simulink model "rtwdemo_pmsmfoc_nn"  (Simulink 7.9)
settings: Solver=FixedStepDiscrete  SolverMode=SingleTasking  StartTime=0.0  StopTime=0.14  FixedStep=ctrlConst.TsHi  RelTol=1e-3
PreLoadFcn:
  | rtwdemo_pmsmfoc_data
undefined symbols (not defined in the file or in its folder): ctrlConst, ctrlParams, DiscIntNeverNeededParam, EnumControllerMode, EnumErrorType
libraries: simulink x15
(part 1 of 2)
Description:
  | Controller Algorithm for Permanent Magnet Synchronous Machine
  | 
  | Specifies controller software component for Permanent Magnet Synchronous Machine (PMSM) using Field-Oriented Control.
  | The sensors bus/structure contains values returned by the Analog to Digital Converter (ADC) and quadrature encoder peripherals.
  | The controller outputs compare values used by the Pulse Width Modulators (PWMs) to generate the phase voltages.
settings Model: MinMaxOverflowLogging=ForceOff  Creator=The MathWorks Inc.  LastModifiedBy=bas  CovHTMLOptions=-aTS=1 -bRG=1 -bTC=1 -hTR=0 -nFC=0 -scm=1 -bcm=1 -xEv=0
settings DataIOCC: ExternalInput=in.motor_on in.command_type in.command_value in.sensors  LimitDataPoints=off  SaveFormat=StructureWithTime  SaveOutput=off  DSMLogging=off  SaveTime=off
settings OptimizationCC: InlineParams=on  UseFloatMulNetSlope=on  UseSpecifiedMinMax=on  InlineInvariantSignals=on  EnhancedBackFolding=on  StrengthReduction=on  ZeroExternalMemoryAtStartup=off  EfficientFloat2IntCast=on  OptimizeModelRefInitCode=on  LifeSpan=1  SimCompilerOptimization=On
settings DebuggingCC: AlgebraicLoopMsg=none  SolverPrmCheckMsg=none  SingleTaskRateTransMsg=error  IntegerOverflowMsg=none  ParameterPrecisionLossMsg=none  UniqueDataStoreMsg=error  AssertControl=DisableAll  ModelReferenceSymbolNameMessage=none
settings HardwareCC: ProdEndianess=LittleEndian  ProdHWDeviceType=Generic->32-bit Embedded Processor
settings ModelReferenceCC: ModelReferenceNumInstancesAllowed=Single
settings RTWCC: SystemTargetFile=nanonote.tlc  TemplateMakefile=nanonote.tmf  Description=Ben NanoNote  GenerateReport=on  RTWVerbose=off  ProcessScript=nanonote_make_rtw_hook  IncludeHyperlinkInReport=on  LaunchReport=on  GenerateTraceInfo=on  GenerateTraceReport=on  GenerateTraceReportSl=on  GenerateTraceReportSf=on  GenerateTraceReportEml=on  GenerateCodeMetricsReport=on  RTWCompilerOptimization=On
settings CodeAppCC: IgnoreCustomStorageClasses=off  IgnoreTestpoints=on  MATLABFcnDesc=on  CustomSymbolStrGlobalVar=$N$M  CustomSymbolStrType=$N$M  CustomSymbolStrFcn=$N$M$F  CustomSymbolStrFcnArg=$N$M  CustomSymbolStrBlkIO=$N$M  CustomSymbolStrMacro=$N$M  MATLABSourceComments=on  ReqsInCode=on
settings STFCustomTargetCC: CodeReplacementLibrary=ANSI_C  CombineOutputUpdateFcns=on  ERTCustomFileBanners=on  SupportContinuousTime=off  SupportNonInlinedSFcns=off  GRTInterface=off  SystemTargetFile=nanonote.tlc
settings ERTTargetCC: CodeReplacementLibrary=ANSI_C  MultiwordLength=2048  ParMdlRefBuildCompliant=off  CompOptLevelCompliant=off  ConcurrentExecutionCompliant=off  ERTFirstTimeCompliant=off  ModelStepFunctionPrototypeControlCompliant=off  CPPClassGenCompliant=off  InlinedParameterPlacement=NonHierarchical  ERTCustomFileTemplate=nanonote_srmain.tlc  ConvertIfToSwitch=off  SuppressUnreachableDefaultCases=off
settings CustomProperty: Value=on
settings ConfigurationSet: Description=SimMechanics 2G
settings ConfigComp: Description=Design Verifier Custom Configuration Component  DVMode=DesignErrorDetection  DVOutputDir=Work/sldv_output/$ModelName$  DVMaxTestCaseSteps=500  DVTestSuiteOptimization=CombinedObjectives (Nonlinear Extended)  DVDesignMinMaxCheck=on  DVSaveReport=on

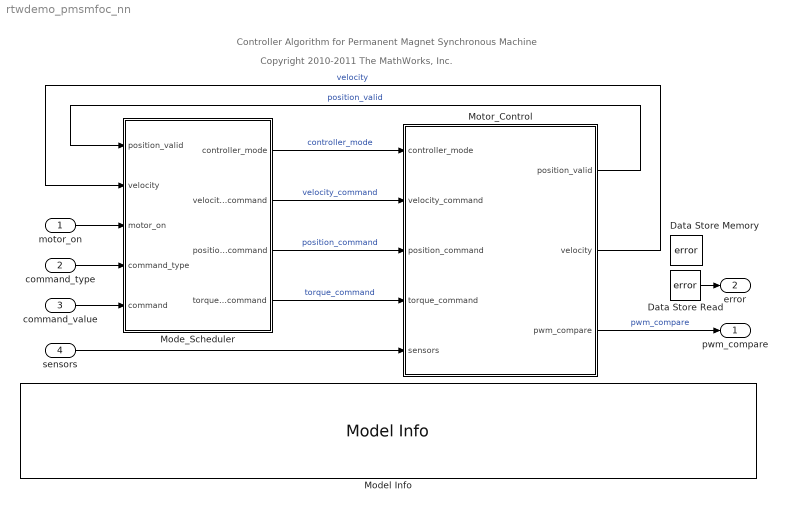
== system rtwdemo_pmsmfoc_nn ==
  note: Controller Algorithm for Permanent Magnet Synchronous Machine
  note: Copyright 2010-2011 The MathWorks, Inc.
  motor_on : Inport  OutDataTypeStr=uint16
  command_type : Inport  Port=2  OutDataTypeStr=Enum: EnumCommandType  Interpolate=off
  command_value : Inport  Port=3  OutDataTypeStr=single  Interpolate=off
  sensors : Inport  Port=4  OutDataTypeStr=Bus: SENSORS_STRUCT  PortDimensions=1  SampleTime=ctrlConst.TsHi  Interpolate=off  BusOutputAsStruct=on
  Data Store Memory : DataStoreMemory  DataStoreName=error  WriteAfterWriteMsg=warning  InitialValue=EnumErrorType.NoError  OutDataTypeStr=Enum: EnumErrorType
  Data Store Read : DataStoreRead  DataStoreName=error  SampleTime=ctrlConst.TsHi
  Mode_Scheduler : Subsystem
      mask Display: fprintf('Mode\nScheduler')
  Model Info : simulink/Model-Wide Utilities/Model Info  InitialBlockCM=None  BlockCM=None  Frame=on  DisplayStringWithTags=Model Description: %<Description>  HorizontalTextAlignment=Left  LeftAlignmentValue=0.02  SourceBlockDiagram=rtwdemo_pmsmfoc_nn  TagMaxNumber=20
  Motor_Control : Subsystem
      settings: RTWSystemCode=Function  RTWFcnNameOpts=Use subsystem name
      mask Display: fprintf('Motor\nControl')
  pwm_compare : Outport
  error : Outport  Port=2
  wires:
  motor_on/1 -> Mode_Scheduler/3(motor_on)
  sensors/1 -> Motor_Control/5(sensors)
  command_type/1 -> Mode_Scheduler/4(command_type)
  Motor_Control/3(pwm_compare) -> pwm_compare/1  "pwm_compare"
  Motor_Control/1(position_valid) -> Mode_Scheduler/1(position_valid)  "position_valid"
  command_value/1 -> Mode_Scheduler/5(command)
  Mode_Scheduler/1(controller_mode) -> Motor_Control/1(controller_mode)  "controller_mode"
  Mode_Scheduler/2(velocity_command) -> Motor_Control/2(velocity_command)  "velocity_command"
  Mode_Scheduler/3(position_command) -> Motor_Control/3(position_command)  "position_command"
  Mode_Scheduler/4(torque_command) -> Motor_Control/4(torque_command)  "torque_command"
  Motor_Control/2(velocity) -> Mode_Scheduler/2(velocity)  "velocity"
  Data Store Read/1 -> error/1

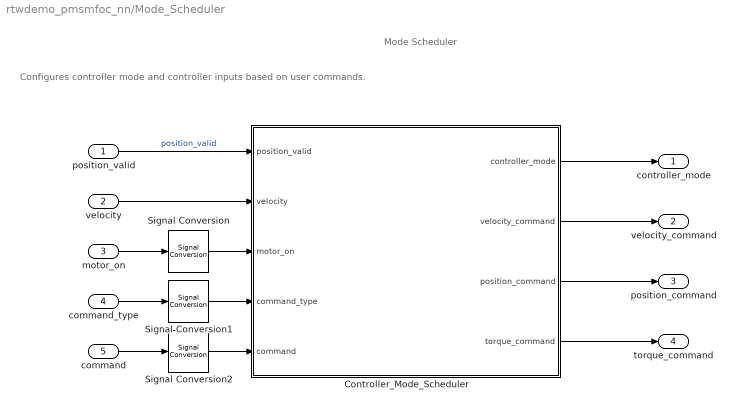
== system rtwdemo_pmsmfoc_nn/Mode_Scheduler ==
  note: Configures controller mode and controller inputs based on user commands.
  note: Mode Scheduler
  position_valid : Inport
  velocity : Inport  Port=2
  motor_on : Inport  Port=3
  command_type : Inport  Port=4
  command : Inport  Port=5
  Controller_Mode_Scheduler : Stateflow chart  TreatAsAtomicUnit=on
  Signal Conversion : SignalConversion  OverrideOpt=on
  Signal Conversion1 : SignalConversion  OverrideOpt=on
  Signal Conversion2 : SignalConversion  OverrideOpt=on
  controller_mode : Outport
  velocity_command : Outport  Port=2
  position_command : Outport  Port=3
  torque_command : Outport  Port=4
  wires:
  position_valid/1 -> Controller_Mode_Scheduler/1(position_valid)  "position_valid"
  Controller_Mode_Scheduler/1(controller_mode) -> controller_mode/1
  velocity/1 -> Controller_Mode_Scheduler/2(velocity)
  Controller_Mode_Scheduler/2(velocity_command) -> velocity_command/1
  motor_on/1 -> Signal Conversion/1
  Controller_Mode_Scheduler/3(position_command) -> position_command/1
  command_type/1 -> Signal Conversion1/1
  Controller_Mode_Scheduler/4(torque_command) -> torque_command/1
  command/1 -> Signal Conversion2/1
  Signal Conversion/1 -> Controller_Mode_Scheduler/3(motor_on)
  Signal Conversion1/1 -> Controller_Mode_Scheduler/4(command_type)
  Signal Conversion2/1 -> Controller_Mode_Scheduler/5(command)

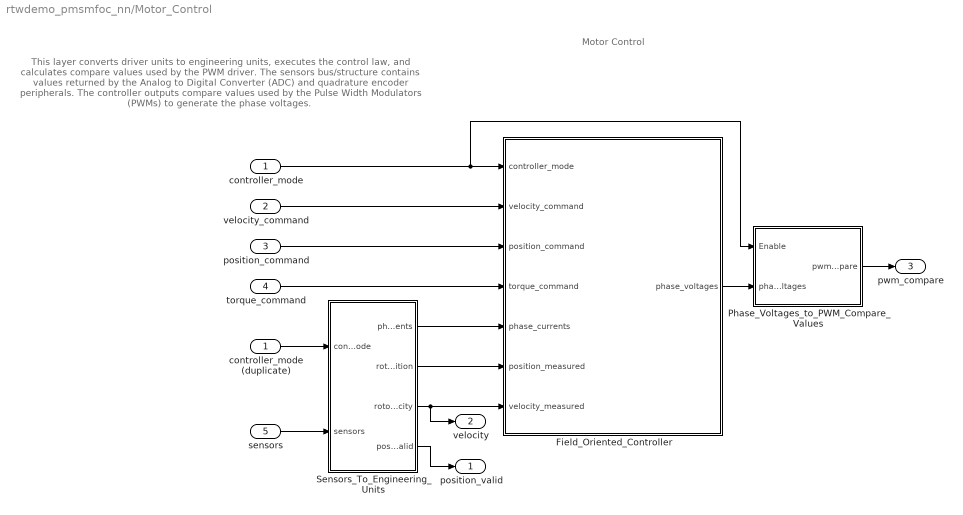
== system rtwdemo_pmsmfoc_nn/Motor_Control ==
  note: This layer converts driver units to engineering units, executes the control law, and calculates compare values used by the PWM driver.
      | The sensors bus/structure contains values returned by the Analog to Digital Converter (ADC) and quadrature encoder peripherals.
      | The controller outputs compare values used by the Pulse Width Modulators (PWMs) to generate the phase voltages.
  note: Motor Control
  controller_mode : Inport
  velocity_command : Inport  Port=2
  position_command : Inport  Port=3
  torque_command : Inport  Port=4
  sensors : Inport  Port=5
  Field_Oriented_Controller : Subsystem
  Phase_Voltages_to_PWM_Compare_Values : Subsystem
      mask Display: fprintf('Phase Voltages\nto PWM\nCompare Values');
  Sensors_To_Engineering_Units : Subsystem
      mask Display: fprintf('Sensors\nto\nEngineering\nUnits')
  controller_mode (duplicate) : InportShadow  Port=1
  position_valid : Outport
  velocity : Outport  Port=2
  pwm_compare : Outport  Port=3
  wires:
  Phase_Voltages_to_PWM_Compare_Values/1(pwm_compare) -> pwm_compare/1
  Field_Oriented_Controller/1(phase_voltages) -> Phase_Voltages_to_PWM_Compare_Values/2(phase_voltages)
  Sensors_To_Engineering_Units/1(phase_currents) -> Field_Oriented_Controller/5(phase_currents)
  controller_mode/1 -> Field_Oriented_Controller/1(controller_mode), Phase_Voltages_to_PWM_Compare_Values/1(Enable)
  sensors/1 -> Sensors_To_Engineering_Units/2(sensors)
  Sensors_To_Engineering_Units/4(position_valid) -> position_valid/1
  Sensors_To_Engineering_Units/3(rotor_velocity) -> velocity/1, Field_Oriented_Controller/7(velocity_measured)
  velocity_command/1 -> Field_Oriented_Controller/2(velocity_command)
  position_command/1 -> Field_Oriented_Controller/3(position_command)
  torque_command/1 -> Field_Oriented_Controller/4(torque_command)
  Sensors_To_Engineering_Units/2(rotor_position) -> Field_Oriented_Controller/6(position_measured)
  controller_mode (duplicate)/1 -> Sensors_To_Engineering_Units/1(controller_mode)

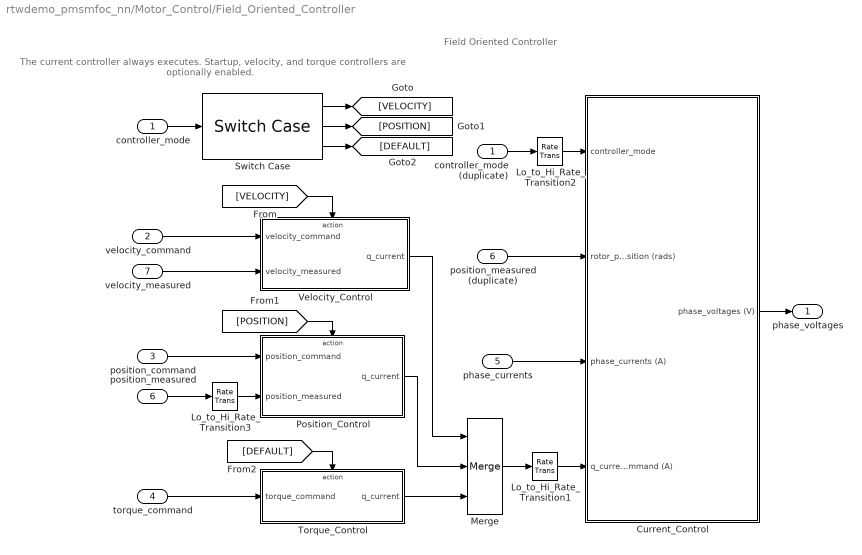
== system rtwdemo_pmsmfoc_nn/Motor_Control/Field_Oriented_Controller ==
  note: The current controller always executes. Startup, velocity, and torque controllers are optionally enabled.
  note: Field Oriented Controller
  controller_mode : Inport
  velocity_command : Inport  Port=2
  position_command : Inport  Port=3
  torque_command : Inport  Port=4
  phase_currents : Inport  Port=5
  position_measured : Inport  Port=6
  velocity_measured : Inport  Port=7
  Current_Control : Subsystem
  Lo_to_Hi_Rate_Transition1 : RateTransition  Integrity=off  OutPortSampleTimeMultiple=25  OutPortSampleTime=ctrlConst.TsHi
  Lo_to_Hi_Rate_Transition2 : RateTransition  Integrity=off  OutPortSampleTimeMultiple=25  OutPortSampleTime=ctrlConst.TsHi
  Lo_to_Hi_Rate_Transition3 : RateTransition  Integrity=off  OutPortSampleTimeMultiple=25  OutPortSampleTime=ctrlConst.TsLo
  Merge : Merge  Inputs=3
  Position_Control : Subsystem  TreatAsAtomicUnit=on
  Switch Case : SwitchCase  CaseConditions={EnumControllerMode.VelocityControl,EnumControllerMode.PositionControl}
  Torque_Control : Subsystem  TreatAsAtomicUnit=on
  Velocity_Control : Subsystem
  controller_mode (duplicate) : InportShadow  Port=1
  position_measured (duplicate) : InportShadow  Port=6
  phase_voltages : Outport
  wires:
  Current_Control/1(phase_voltages (V)) -> phase_voltages/1
  velocity_measured/1 -> Velocity_Control/2(velocity_measured)
  Position_Control/1(q_current) -> Merge/2
  Velocity_Control/1(q_current) -> Merge/1
  Torque_Control/1(q_current) -> Merge/3
  controller_mode/1 -> Switch Case/1
  Merge/1 -> Lo_to_Hi_Rate_Transition1/1
  phase_currents/1 -> Current_Control/3(phase_currents (A))
  controller_mode (duplicate)/1 -> Lo_to_Hi_Rate_Transition2/1
  velocity_command/1 -> Velocity_Control/1(velocity_command)
  position_measured (duplicate)/1 -> Current_Control/2(rotor_position (rads))
  torque_command/1 -> Torque_Control/1(torque_command)
  position_command/1 -> Position_Control/1(position_command)
  position_measured/1 -> Lo_to_Hi_Rate_Transition3/1
  Switch Case/1 -> [VELOCITY]
  Switch Case/2 -> [POSITION]
  Switch Case/3 -> [DEFAULT]
  [VELOCITY] -> Velocity_Control/Action
  [POSITION] -> Position_Control/Action
  [DEFAULT] -> Torque_Control/Action
  Lo_to_Hi_Rate_Transition3/1 -> Position_Control/2(position_measured)
  Lo_to_Hi_Rate_Transition1/1 -> Current_Control/4(q_current_command (A))
  Lo_to_Hi_Rate_Transition2/1 -> Current_Control/1(controller_mode)

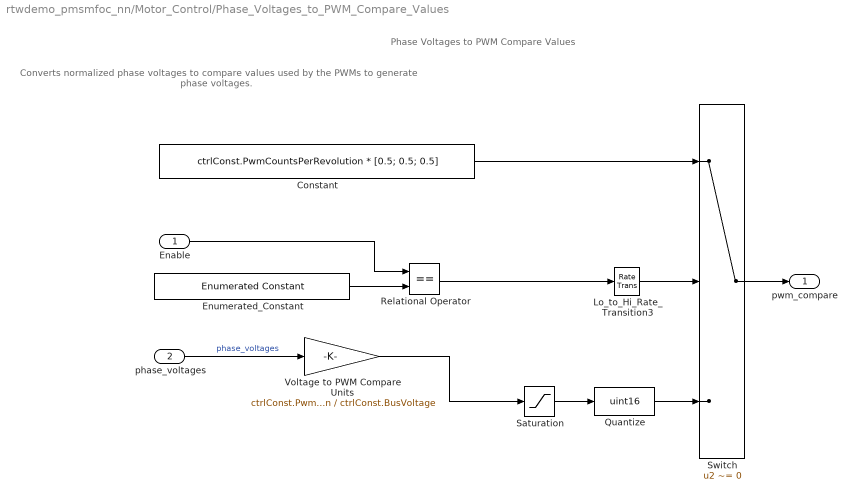
== system rtwdemo_pmsmfoc_nn/Motor_Control/Phase_Voltages_to_PWM_Compare_Values ==
  note: Converts normalized phase voltages to compare values used by the PWMs to generate phase voltages.
  note: Phase Voltages to PWM Compare Values
  Enable : Inport
  phase_voltages : Inport  Port=2
  Constant : Constant  Value=ctrlConst.PwmCountsPerRevolution * [0.5; 0.5; 0.5]  OutDataTypeStr=uint16
  Enumerated_Constant : simulink/Sources/Enumerated Constant  OutDataTypeStr=Enum: EnumControllerMode  Value=EnumControllerMode.StandBy  SampleTime=inf
  Lo_to_Hi_Rate_Transition3 : RateTransition  Deterministic=off  OutPortSampleTimeMultiple=25  OutPortSampleTime=ctrlConst.TsHi
      settings: AttributesFormatString=------------------\nSample Time:\n%<OutPortSampleTime>
  Quantize : DataTypeConversion  OutDataTypeStr=uint16  RndMeth=Simplest
  Relational Operator : RelationalOperator  Operator===  OutDataTypeStr=boolean
  Saturation : Saturate  UpperLimit=ctrlConst.PwmCountsPerRevolution - 1  LowerLimit=0
      settings: AttributesFormatString=--------------------------------\nUpper Limit: %<UpperLimit>\nLower Limit: %<LowerLimit>
  Switch : Switch  Criteria=u2 ~= 0
  Voltage to PWM Compare Units : Gain  Gain=ctrlConst.PwmCountsPerRevolution / ctrlConst.BusVoltage
      settings: AttributesFormatString=----------------------------------------\nGain:\n%<Gain>
  pwm_compare : Outport
  wires:
  phase_voltages/1 -> Voltage to PWM Compare Units/1  "phase_voltages"
  Voltage to PWM Compare Units/1 -> Saturation/1
  Switch/1 -> pwm_compare/1
  Lo_to_Hi_Rate_Transition3/1 -> Switch/2
  Enumerated_Constant/1 -> Relational Operator/2
  Enable/1 -> Relational Operator/1
  Relational Operator/1 -> Lo_to_Hi_Rate_Transition3/1
  Constant/1 -> Switch/1
  Saturation/1 -> Quantize/1
  Quantize/1 -> Switch/3

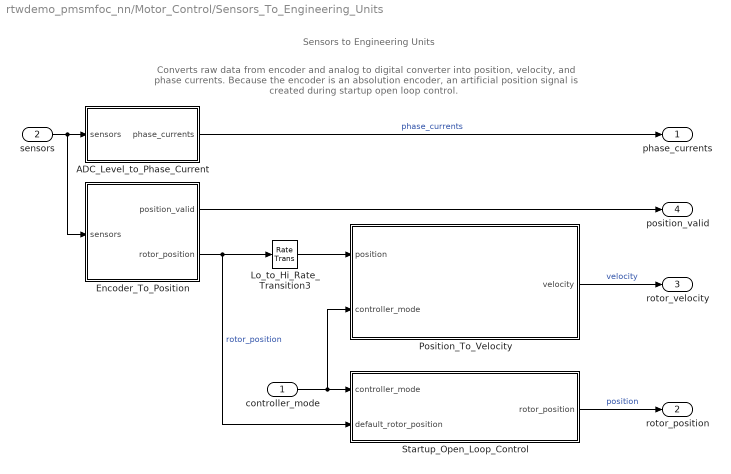
== system rtwdemo_pmsmfoc_nn/Motor_Control/Sensors_To_Engineering_Units ==
  note: Sensors to Engineering Units
  note: Converts raw data from encoder and analog to digital converter into position, velocity, and phase currents.
      | Because the encoder is an absolution encoder, an artificial position signal is created during startup open loop control.
  controller_mode : Inport
  sensors : Inport  Port=2
  ADC_Level_to_Phase_Current : Subsystem
      mask Display: fprintf('ADC Level\nto\nPhase Currents')
  Encoder_To_Position : Subsystem
      mask Display: fprintf('Encoder\nto\nPosition')
  Lo_to_Hi_Rate_Transition3 : RateTransition  Integrity=off  OutPortSampleTimeMultiple=25  OutPortSampleTime=ctrlConst.TsLo
      settings: AttributesFormatString=------------------\nSample Time:\n%<OutPortSampleTime>
  Position_To_Velocity : Subsystem  Variant=on  OverrideUsingVariant=IMPLICIT_WITH_ERROR
  Startup_Open_Loop_Control : Subsystem
      mask Display: fprintf('Startup\nOpen Loop\nControl')
  phase_currents : Outport
  rotor_position : Outport  Port=2
  rotor_velocity : Outport  Port=3
  position_valid : Outport  Port=4
  wires:
  ADC_Level_to_Phase_Current/1(phase_currents) -> phase_currents/1  "phase_currents"
  sensors/1 -> ADC_Level_to_Phase_Current/1(sensors), Encoder_To_Position/1(sensors)
  Position_To_Velocity/1(velocity) -> rotor_velocity/1  "velocity"
  Lo_to_Hi_Rate_Transition3/1 -> Position_To_Velocity/1(position)
  Startup_Open_Loop_Control/1(rotor_position) -> rotor_position/1  "position"
  controller_mode/1 -> Startup_Open_Loop_Control/1(controller_mode), Position_To_Velocity/2(controller_mode)
  Encoder_To_Position/1(position_valid) -> position_valid/1
  Encoder_To_Position/2(rotor_position) -> Startup_Open_Loop_Control/2(default_rotor_position), Lo_to_Hi_Rate_Transition3/1  "rotor_position"

== system rtwdemo_pmsmfoc_nn/Motor_Control/Field_Oriented_Controller/Current_Control ==
  note: Controls stator currents based on transformations between a three-phase phase time and speed dependent system (ABC)
      | and a two coordinate time invariant system (dq).
  note: Current Control
  controller_mode : Inport
  rotor_position (rads) : Inport  Port=2
  phase_currents (A) : Inport  Port=3
  q_current_command (A) : Inport  Port=4
  Current_Controllers : Subsystem  Description=|
      | Linear Current Controllers
      | 
      | PID Blocks used for Control Design of Current Loop controllers.
  Detect_Change : simulink/Logic and Bit Operations/Detect Change  vinit=0  InputProcessing=Inherited  OutDataTypeStr=uint8
  Enum_To_Int : DataTypeConversion  OutDataTypeStr=int16
  Rotation_Coefficients_Sin_Cos : Subsystem
      mask Display: disp('Rotation\nCoefficients\n(sin, cos)')
  Transform_Coordinates_ABC_to_dq : Subsystem
      settings: RTWSystemCode=Function
      mask Display: disp('Transform\nCoordinates\nABC to dq')
  Transform_Coordinates_dq_to_ABC : Subsystem
      settings: RTWSystemCode=Function
      mask Display: disp('Transform\nCoordinates\ndq to ABC')
  phase_voltages (V) : Outport
  wires:
  Current_Controllers/1(dq_axis_voltages (V)) -> Transform_Coordinates_dq_to_ABC/1(dq_voltages)
  phase_currents (A)/1 -> Transform_Coordinates_ABC_to_dq/1(phase_currents)
  Rotation_Coefficients_Sin_Cos/1(sin_cos) -> Transform_Coordinates_dq_to_ABC/2(rotation_coefficients), Transform_Coordinates_ABC_to_dq/2(rotation_coefficients)
  Transform_Coordinates_dq_to_ABC/1(phase_voltages) -> phase_voltages (V)/1
  Transform_Coordinates_ABC_to_dq/1(d_current) -> Current_Controllers/3(d_current_measured (A))
  controller_mode/1 -> Enum_To_Int/1
  rotor_position (rads)/1 -> Rotation_Coefficients_Sin_Cos/1(rotor_position)
  q_current_command (A)/1 -> Current_Controllers/2(q_current_command (A))
  Transform_Coordinates_ABC_to_dq/2(q_current) -> Current_Controllers/4(q_current_measured (A))
  Detect_Change/1 -> Current_Controllers/1(reset_integrators)
  Enum_To_Int/1 -> Detect_Change/1

== system rtwdemo_pmsmfoc_nn/Motor_Control/Field_Oriented_Controller/Position_Control ==
  note: The controller regulates motor position using rotor position feedback compared to a commanded position.
      | The output of the controller is the quadrature-winding current command which is directly proportional to the electromagnetic torque of the motor.
      | Since the motor being controlled is a Permanent Magnet Synchronous Machine, the rotor flux linkage is fixed (determined by the magnets),
      | hence the commanded direct-winding current is always zero.
  note: Position Controller
  position_command : Inport
  position_measured : Inport  Port=2
  Action Port : ActionPort  InitializeStates=reset  ActionType=case
      settings: AttributesFormatString=----------------------------\nStates: %<InitializeStates>
  Isolate_For_Merge : SignalConversion
  Position_Control : simulink/Continuous/PID Controller  Controller=PI  TimeDomain=Discrete-time  SampleTime=-1  IntegratorMethod=Forward Euler  FilterMethod=Forward Euler  Form=Parallel  P=ctrlParams.Position_P  I=ctrlParams.Position_I  D=0  N=100  InitialConditionSource=internal  InitialConditionForIntegrator=0  InitialConditionForFilter=0  ExternalReset=none  LimitOutput=on  UpperSaturationLimit=ctrlConst.CurrentLimit  LowerSaturationLimit=-ctrlConst.CurrentLimit  LinearizeAsGain=off  AntiWindupMode=clamping  Kb=0  TrackingMode=off  Kt=1  PParamMin=[]  PParamMax=[]  IParamMin=[]  IParamMax=[]  DParamMin=[]  DParamMax=[]  NParamMin=[]  NParamMax=[]  KbParamMin=[]  KbParamMax=[]  KtParamMin=[]  KtParamMax=[]  POutMin=[]  POutMax=[]  IOutMin=[]  IOutMax=[]  DOutMin=[]  DOutMax=[]  NOutMin=[]  NOutMax=[]  KbOutMin=[]  KbOutMax=[]  KtOutMin=[]  KtOutMax=[]  IntegratorOutMin=[]  IntegratorOutMax=[]  FilterOutMin=[]  FilterOutMax=[]  SumOutMin=[]  SumOutMax=[]  SumI1OutMin=[]  SumI1OutMax=[]  SumI2OutMin=[]  SumI2OutMax=[]  SumI3OutMin=[]  SumI3OutMax=[]  SumDOutMin=[]  SumDOutMax=[]  SaturationOutMin=[]  SaturationOutMax=[]  IntegratorContinuousStateAttributes=''  IntegratorStateMustResolveToSignalObject=off  IntegratorRTWStateStorageClass=Auto  FilterContinuousStateAttributes=''  FilterStateMustResolveToSignalObject=off  FilterRTWStateStorageClass=Auto
      settings: AttributesFormatString=-----------------------------------\nP Gain: %<P>\nI Gain: %<I>
  Sum2 : Sum  Inputs=|+-
  Wrap_Error_pi : Subsystem
  q_current : Outport
  wires:
  position_measured/1 -> Sum2/2  "position_measured"
  position_command/1 -> Sum2/1  "position_command"
  Position_Control/1 -> Isolate_For_Merge/1  "quadrature_current_command"
  Sum2/1 -> Wrap_Error_pi/1(Error)  "position_error"
  Wrap_Error_pi/1(Wrap) -> Position_Control/1  "position_error_wrap"
  Isolate_For_Merge/1 -> q_current/1

== system rtwdemo_pmsmfoc_nn/Motor_Control/Field_Oriented_Controller/Torque_Control ==
  note: The output of the controller is the quadrature-winding current command which is directly proportional to the electromagnetic torque of the motor.
      | In this configuration, the torque command is just the current command. An additional gain term could be added to translate current to torque
      | based on know motor parameters.
  note: Torque Controller
  torque_command : Inport
  Action Port : ActionPort  ActionType=default
      settings: AttributesFormatString=----------------------------\nStates: %<InitializeStates>
  q_current : Outport
  wires:
  torque_command/1 -> q_current/1

== system rtwdemo_pmsmfoc_nn/Motor_Control/Field_Oriented_Controller/Velocity_Control ==
  note: The controller regulates motor velocity using rotor velocity feedback compared to a commanded velocity.
      | The output of the controller is the quadrature-winding current command which is directly proportional to the electromagnetic torque of the motor.
      | Since the motor being controlled is a Permanent Magnet Synchronous Machine, the rotor flux linkage is fixed (determined by the magnets),
      | hence the commanded direct-winding current is always zero.
  note: Velocity Controller
  velocity_command : Inport
  velocity_measured : Inport  Port=2
  Action Port : ActionPort  InitializeStates=reset  ActionType=case
      settings: AttributesFormatString=----------------------------\nStates: %<InitializeStates>
  Isolate_For_Merge : SignalConversion
  Rotor_Speed_Control : simulink/Continuous/PID Controller  Controller=PI  TimeDomain=Discrete-time  SampleTime=-1  IntegratorMethod=Forward Euler  FilterMethod=Forward Euler  Form=Parallel  P=ctrlParams.Velocity_P  I=ctrlParams.Velocity_I  D=0  N=100  InitialConditionSource=internal  InitialConditionForIntegrator=0  InitialConditionForFilter=0  ExternalReset=none  LimitOutput=on  UpperSaturationLimit=ctrlConst.CurrentLimit  LowerSaturationLimit=-ctrlConst.CurrentLimit  LinearizeAsGain=off  AntiWindupMode=clamping  Kb=0  TrackingMode=off  Kt=1  PParamMin=[]  PParamMax=[]  IParamMin=[]  IParamMax=[]  DParamMin=[]  DParamMax=[]  NParamMin=[]  NParamMax=[]  KbParamMin=[]  KbParamMax=[]  KtParamMin=[]  KtParamMax=[]  POutMin=[]  POutMax=[]  IOutMin=[]  IOutMax=[]  DOutMin=[]  DOutMax=[]  NOutMin=[]  NOutMax=[]  KbOutMin=[]  KbOutMax=[]  KtOutMin=[]  KtOutMax=[]  IntegratorOutMin=[]  IntegratorOutMax=[]  FilterOutMin=[]  FilterOutMax=[]  SumOutMin=[]  SumOutMax=[]  SumI1OutMin=[]  SumI1OutMax=[]  SumI2OutMin=[]  SumI2OutMax=[]  SumI3OutMin=[]  SumI3OutMax=[]  SumDOutMin=[]  SumDOutMax=[]  SaturationOutMin=[]  SaturationOutMax=[]  IntegratorContinuousStateAttributes=''  IntegratorStateMustResolveToSignalObject=off  IntegratorRTWStateStorageClass=Auto  FilterContinuousStateAttributes=''  FilterStateMustResolveToSignalObject=off  FilterRTWStateStorageClass=Auto
      settings: AttributesFormatString=----------------------------------------------\nP Gain: %<P>\nI Gain: %<I>
  Sum2 : Sum  Inputs=|+-
  q_current : Outport
  wires:
  velocity_measured/1 -> Sum2/2  "velocity_measured"
  Sum2/1 -> Rotor_Speed_Control/1  "velocity_error"
  Rotor_Speed_Control/1 -> Isolate_For_Merge/1  "quadrature_current_command"
  velocity_command/1 -> Sum2/1  "velocity_command"
  Isolate_For_Merge/1 -> q_current/1

== system rtwdemo_pmsmfoc_nn/Motor_Control/Sensors_To_Engineering_Units/ADC_Level_to_Phase_Current ==
  note: Calculate phase current in Amps from integer result returned by analog to digital converter.
  note: ADC Level to Phase Current
  sensors : Inport
  ADC_Driver_Units_To_Amps : Constant  Value=ctrlParams.AdcDriverUnitsToAmps
  ADC_Zero_Offset : Constant  Value=ctrlParams.AdcZeroOffsetDriverUnits
  Add : Sum  Inputs=+-
  Bus Selector : BusSelector  OutputSignals=adc_phase_currents
  Product : Product  RndMeth=Zero
  phase_currents : Outport
  wires:
  sensors/1 -> Bus Selector/1
  Bus Selector/1 -> Add/1  "<adc_phase_currents>"
  ADC_Zero_Offset/1 -> Add/2
  Add/1 -> Product/1
  ADC_Driver_Units_To_Amps/1 -> Product/2
  Product/1 -> phase_currents/1

== system rtwdemo_pmsmfoc_nn/Motor_Control/Sensors_To_Engineering_Units/Encoder_To_Position ==
  note: The encoder counts increase with positive rotation of the rotor.
  note: Encoder to Position
  sensors : Inport
  Add : Sum
  Bus Selector : BusSelector  OutputSignals=encoder_counter,encoder_valid
  Lo_to_Hi_Rate_Transition1 : RateTransition  Integrity=off  Deterministic=off  OutPortSampleTimeMultiple=25  OutPortSampleTime=ctrlConst.TsLo
      settings: AttributesFormatString=------------------\nSample Time:\n%<OutPortSampleTime>
  Offset_Between_Encoder_Zero_And_Mechanical_Zero : Constant  Value=ctrlParams.EncoderToMechanicalZeroOffsetRads  OutDataTypeStr=single
  Wait_For_Valid_Position : Stateflow chart
  radians_per_counts : Gain  Gain=2*pi / ctrlConst.EncoderCountsPerRevolution  ParamDataTypeStr=single  OutDataTypeStr=single
      settings: AttributesFormatString=---------------------------------------------------\nGain: %<Gain>
  position_valid : Outport
  rotor_position : Outport  Port=2
  wires:
  sensors/1 -> Bus Selector/1
  Bus Selector/1 -> radians_per_counts/1  "<encoder_counter>"
  Wait_For_Valid_Position/1(Position_Valid) -> Lo_to_Hi_Rate_Transition1/1
  Bus Selector/2 -> Wait_For_Valid_Position/1(encoder_valid)  "<encoder_valid>"
  Lo_to_Hi_Rate_Transition1/1 -> position_valid/1
  Add/1 -> rotor_position/1  "rotor_angle"
  Offset_Between_Encoder_Zero_And_Mechanical_Zero/1 -> Add/1
  radians_per_counts/1 -> Add/2  "encoder_angle"

== system rtwdemo_pmsmfoc_nn/Motor_Control/Sensors_To_Engineering_Units/Position_To_Velocity ==
  note: 1) Only subsystems can be added as variant choices at this level
      | 2) Blocks cannot be connected at this level as connectivity is
      | automatically determined at simulation, based on the active variant
  note: Velocity Calculation Variant Subsystem
  note: Specifies different methods to calculate velocity.
      | Ports are connected based on the active variant for this subsystem.
  position : Inport
  controller_mode : Inport  Port=2
  Explicit_Angle_Wrap : Subsystem  VariantObject=EXPLICIT
      settings: RTWSystemCode=Function
  Explicit_Angle_Wrap_With_Error : Subsystem  VariantObject=EXPLICIT_WITH_ERROR
      settings: RTWSystemCode=Function
  Implicit_Integer_Wrap_With_Error : Subsystem  VariantObject=IMPLICIT_WITH_ERROR
      settings: RTWSystemCode=Function
  velocity : Outport

== system rtwdemo_pmsmfoc_nn/Motor_Control/Sensors_To_Engineering_Units/Startup_Open_Loop_Control ==
  note: Startup Open Loop Control
  note: Generates artificial position when in Startup mode, else passes the measured rotor position.
  controller_mode : Inport
  default_rotor_position : Inport  Port=2
  Enumerated Constant : simulink/Sources/Enumerated Constant  OutDataTypeStr=Enum: EnumControllerMode  Value=EnumControllerMode.Startup  SampleTime=inf
  Lo_to_Hi_Rate_Transition2 : RateTransition  Integrity=off  Deterministic=off  OutPortSampleTimeMultiple=25  OutPortSampleTime=ctrlConst.TsHi
      settings: AttributesFormatString=------------------\nSample Time:\n%<OutPortSampleTime>
  Open Loop Position : Subsystem
  Relational Operator : RelationalOperator  Operator===  OutDataTypeStr=boolean
  Switch : Switch  Criteria=u2 ~= 0
  rotor_position : Outport
  wires:
  default_rotor_position/1 -> Switch/3
  Switch/1 -> rotor_position/1
  Open Loop Position/1(rotor_position) -> Switch/1
  Lo_to_Hi_Rate_Transition2/1 -> Open Loop Position/Enable, Switch/2
  Enumerated Constant/1 -> Relational Operator/2
  controller_mode/1 -> Relational Operator/1
  Relational Operator/1 -> Lo_to_Hi_Rate_Transition2/1

== system rtwdemo_pmsmfoc_nn/Motor_Control/Field_Oriented_Controller/Current_Control/Current_Controllers ==
  note: Current Controllers
  note: The controller regulates direct and quadrature currents.
  reset_integrators : Inport
  q_current_command (A) : Inport  Port=2
  d_current_measured (A) : Inport  Port=3
  q_current_measured (A) : Inport  Port=4
  Bus Creator : BusCreator  Inputs=2
  Direct_Current_Control : simulink/Continuous/PID Controller  Controller=PI  TimeDomain=Discrete-time  SampleTime=-1  IntegratorMethod=Forward Euler  FilterMethod=Forward Euler  Form=Parallel  P=ctrlParams.Current_P  I=ctrlParams.Current_I  D=0  N=100  InitialConditionSource=internal  InitialConditionForIntegrator=0  InitialConditionForFilter=0  ExternalReset=level  LimitOutput=on  UpperSaturationLimit=ctrlConst.VoltageLimit  LowerSaturationLimit=-ctrlConst.VoltageLimit  LinearizeAsGain=off  AntiWindupMode=clamping  Kb=0  TrackingMode=off  Kt=1  PParamMin=[]  PParamMax=[]  IParamMin=[]  IParamMax=[]  DParamMin=[]  DParamMax=[]  NParamMin=[]  NParamMax=[]  KbParamMin=[]  KbParamMax=[]  KtParamMin=[]  KtParamMax=[]  POutMin=[]  POutMax=[]  IOutMin=[]  IOutMax=[]  DOutMin=[]  DOutMax=[]  NOutMin=[]  NOutMax=[]  KbOutMin=[]  KbOutMax=[]  KtOutMin=[]  KtOutMax=[]  IntegratorOutMin=[]  IntegratorOutMax=[]  FilterOutMin=[]  FilterOutMax=[]  SumOutMin=[]  SumOutMax=[]  SumI1OutMin=[]  SumI1OutMax=[]  SumI2OutMin=[]  SumI2OutMax=[]  SumI3OutMin=[]  SumI3OutMax=[]  SumDOutMin=[]  SumDOutMax=[]  SaturationOutMin=[]  SaturationOutMax=[]  IntegratorContinuousStateAttributes=''  IntegratorStateMustResolveToSignalObject=off  IntegratorRTWStateStorageClass=Auto  FilterContinuousStateAttributes=''  FilterStateMustResolveToSignalObject=off  FilterRTWStateStorageClass=Auto
      settings: AttributesFormatString=----------------------------------------------\nP Gain: %<P>\nI Gain: %<I>
  Quadrature_Current_Control : simulink/Continuous/PID Controller  Controller=PI  TimeDomain=Discrete-time  SampleTime=-1  IntegratorMethod=Forward Euler  FilterMethod=Forward Euler  Form=Parallel  P=ctrlParams.Current_P  I=ctrlParams.Current_I  D=0  N=100  InitialConditionSource=internal  InitialConditionForIntegrator=0  InitialConditionForFilter=0  ExternalReset=level  LimitOutput=on  UpperSaturationLimit=ctrlConst.VoltageLimit  LowerSaturationLimit=-ctrlConst.VoltageLimit  LinearizeAsGain=off  AntiWindupMode=clamping  Kb=0  TrackingMode=off  Kt=1  PParamMin=[]  PParamMax=[]  IParamMin=[]  IParamMax=[]  DParamMin=[]  DParamMax=[]  NParamMin=[]  NParamMax=[]  KbParamMin=[]  KbParamMax=[]  KtParamMin=[]  KtParamMax=[]  POutMin=[]  POutMax=[]  IOutMin=[]  IOutMax=[]  DOutMin=[]  DOutMax=[]  NOutMin=[]  NOutMax=[]  KbOutMin=[]  KbOutMax=[]  KtOutMin=[]  KtOutMax=[]  IntegratorOutMin=[]  IntegratorOutMax=[]  FilterOutMin=[]  FilterOutMax=[]  SumOutMin=[]  SumOutMax=[]  SumI1OutMin=[]  SumI1OutMax=[]  SumI2OutMin=[]  SumI2OutMax=[]  SumI3OutMin=[]  SumI3OutMax=[]  SumDOutMin=[]  SumDOutMax=[]  SaturationOutMin=[]  SaturationOutMax=[]  IntegratorContinuousStateAttributes=''  IntegratorStateMustResolveToSignalObject=off  IntegratorRTWStateStorageClass=Auto  FilterContinuousStateAttributes=''  FilterStateMustResolveToSignalObject=off  FilterRTWStateStorageClass=Auto
      settings: AttributesFormatString=----------------------------------------------\nP Gain: %<P>\nI Gain: %<I>
  Sum : Sum  Inputs=|+-
  Sum2 : Sum  Inputs=|+-
  d_current_command (A) : Constant  Value=0  OutDataTypeStr=single
  dq_axis_voltages (V) : Outport
  wires:
  d_current_command (A)/1 -> Sum2/1  "d_current_command"
  Bus Creator/1 -> dq_axis_voltages (V)/1
  q_current_command (A)/1 -> Sum/1  "q_current_command"
  Direct_Current_Control/1 -> Bus Creator/1  "direct_voltage"
  Quadrature_Current_Control/1 -> Bus Creator/2  "quadrature_voltage"
  Sum2/1 -> Direct_Current_Control/1  "d_current_error"
  Sum/1 -> Quadrature_Current_Control/1  "q_current_error"
  reset_integrators/1 -> Direct_Current_Control/2, Quadrature_Current_Control/2
  d_current_measured (A)/1 -> Sum2/2  "d_current_measured"
  q_current_measured (A)/1 -> Sum/2  "q_current_measured"

== system rtwdemo_pmsmfoc_nn/Motor_Control/Field_Oriented_Controller/Current_Control/Rotation_Coefficients_Sin_Cos ==
  note: Rotation Coefficients Sin Cos
  note: Calculate sine and cosine of electrical angle.
  rotor_position : Inport
  Bus Creator : BusCreator  Inputs=2
  number_of_pole_pairs : Gain  Gain=ctrlParams.PmsmPolePairs
      settings: AttributesFormatString=------------------------------------\nGain: %<Gain>
  sine_cosine : Trigonometry  Operator=sincos
  sin_cos : Outport
  wires:
  Bus Creator/1 -> sin_cos/1
  rotor_position/1 -> number_of_pole_pairs/1  "mechanical_angle"
  sine_cosine/1 -> Bus Creator/1  "sin_coefficient"
  sine_cosine/2 -> Bus Creator/2  "cos_coefficient"
  number_of_pole_pairs/1 -> sine_cosine/1  "electrical_angle"

== system rtwdemo_pmsmfoc_nn/Motor_Control/Field_Oriented_Controller/Current_Control/Transform_Coordinates_ABC_to_dq ==
  note: Transform Coordinates ABC to dq
  note: Transforms from a three-phase time and speed dependent system (ABC) to a two coordinate time invariant system (dq).
  phase_currents : Inport
  rotation_coefficients : Inport  Port=2
  Clarke_Transform : Subsystem
  Park_Transform : Subsystem
  d_current : Outport
  q_current : Outport  Port=2
  wires:
  rotation_coefficients/1 -> Park_Transform/1(rotation_coefficients)
  phase_currents/1 -> Clarke_Transform/1(phase_currents)
  Clarke_Transform/1(alpha_current) -> Park_Transform/2(alpha_current)
  Clarke_Transform/2(beta_current) -> Park_Transform/3(beta_current)
  Park_Transform/1(direct_current) -> d_current/1
  Park_Transform/2(quadrature_current) -> q_current/1

== system rtwdemo_pmsmfoc_nn/Motor_Control/Field_Oriented_Controller/Current_Control/Transform_Coordinates_dq_to_ABC ==
  note: Transform Coordinates dq to ABC
  note: Converts the two coordinate time invariant system (dq) to a three-phase time and speed dependent system (ABC).
  dq_voltages : Inport
  rotation_coefficients : Inport  Port=2
  Alpha_Beta_to_ABC : Subsystem  Variant=on  OverrideUsingVariant=SPACE_VECTOR_MODULATION
  Inverse_Park_Transform : Subsystem
  phase_voltages : Outport
  wires:
  rotation_coefficients/1 -> Inverse_Park_Transform/1(rotation_coefficients)
  dq_voltages/1 -> Inverse_Park_Transform/2(dq_voltages)
  Inverse_Park_Transform/1(alpha_voltage) -> Alpha_Beta_to_ABC/1(alpha_voltage)
  Inverse_Park_Transform/2(beta_voltage) -> Alpha_Beta_to_ABC/2(beta_voltage)
  Alpha_Beta_to_ABC/1(phase_voltages) -> phase_voltages/1

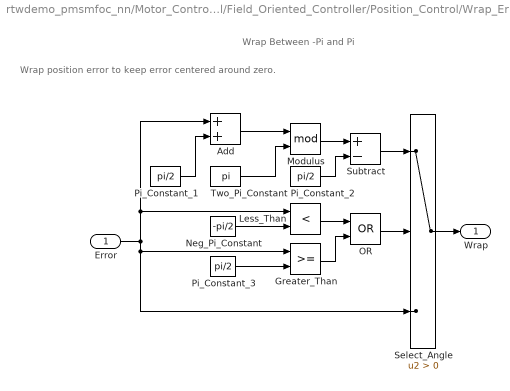
== system rtwdemo_pmsmfoc_nn/Motor_Control/Field_Oriented_Controller/Position_Control/Wrap_Error_pi ==
  note: Wrap position error to keep error centered around zero.
  note: Wrap Between -Pi and Pi
  Error : Inport
  Add : Sum
  Greater_Than : RelationalOperator  OutDataTypeStr=boolean
  Less_Than : RelationalOperator  Operator=<  OutDataTypeStr=boolean
  Modulus : Math  Operator=mod  SaturateOnIntegerOverflow=on
  Neg_Pi_Constant : Constant  Value=-pi/2  OutDataTypeStr=single
  OR : Logic  Operator=OR  AllPortsSameDT=off  OutDataTypeStr=boolean
  Pi_Constant_1 : Constant  Value=pi/2  OutDataTypeStr=single
  Pi_Constant_2 : Constant  Value=pi/2  OutDataTypeStr=single
  Pi_Constant_3 : Constant  Value=pi/2  OutDataTypeStr=single
  Select_Angle : Switch  Criteria=u2 > Threshold
  Subtract : Sum  Inputs=+-
  Two_Pi_Constant : Constant  Value=pi  OutDataTypeStr=single
  Wrap : Outport
  wires:
  Pi_Constant_3/1 -> Greater_Than/2
  Neg_Pi_Constant/1 -> Less_Than/2
  Error/1 -> Select_Angle/3, Greater_Than/1, Add/1, Less_Than/1
  Add/1 -> Modulus/1
  Pi_Constant_1/1 -> Add/2
  Subtract/1 -> Select_Angle/1
  OR/1 -> Select_Angle/2
  Pi_Constant_2/1 -> Subtract/2
  Modulus/1 -> Subtract/1
  Two_Pi_Constant/1 -> Modulus/2
  Greater_Than/1 -> OR/2
  Less_Than/1 -> OR/1
  Select_Angle/1 -> Wrap/1

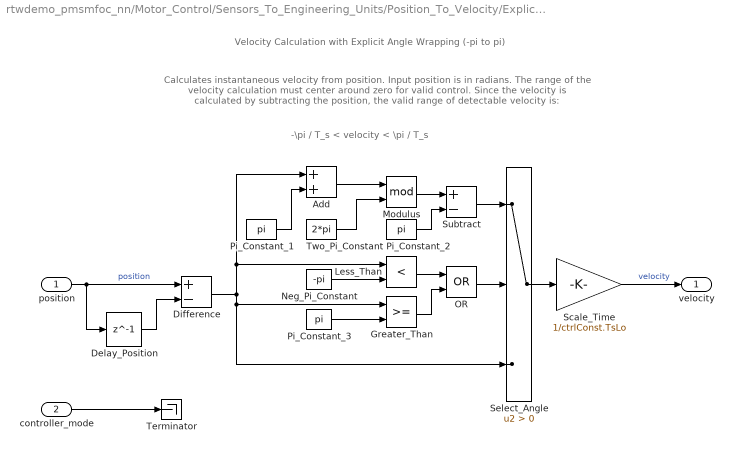
== system rtwdemo_pmsmfoc_nn/Motor_Control/Sensors_To_Engineering_Units/Position_To_Velocity/Explicit_Angle_Wrap ==
  note: Velocity Calculation with Explicit Angle Wrapping (-pi to pi)
  note: Calculates instantaneous velocity from position. Input position is in radians.
      | The range of the velocity calculation must center around zero for valid control.
      | Since the velocity is calculated by subtracting the position, the valid range of detectable velocity is:
  note: -\pi / T_s < velocity < \pi / T_s
  position : Inport
  controller_mode : Inport  Port=2
  Add : Sum
  Delay_Position : Delay  DelayLength=1
  Difference : Sum  Inputs=+-
  Greater_Than : RelationalOperator  OutDataTypeStr=boolean
  Less_Than : RelationalOperator  Operator=<  OutDataTypeStr=boolean
  Modulus : Math  Operator=mod  SaturateOnIntegerOverflow=on
  Neg_Pi_Constant : Constant  Value=-pi  OutDataTypeStr=single
  OR : Logic  Operator=OR  AllPortsSameDT=off  OutDataTypeStr=boolean
  Pi_Constant_1 : Constant  Value=pi  OutDataTypeStr=single
  Pi_Constant_2 : Constant  Value=pi  OutDataTypeStr=single
  Pi_Constant_3 : Constant  Value=pi  OutDataTypeStr=single
  Scale_Time : Gain  Gain=1/ctrlConst.TsLo  OutDataTypeStr=single
      settings: AttributesFormatString=---------------------\n%<Gain>
  Select_Angle : Switch  Criteria=u2 > Threshold
  Subtract : Sum  Inputs=+-
  Terminator : Terminator
  Two_Pi_Constant : Constant  Value=2*pi  OutDataTypeStr=single
  velocity : Outport
  wires:
  Delay_Position/1 -> Difference/2
  position/1 -> Difference/1, Delay_Position/1  "position"
  Less_Than/1 -> OR/1
  Greater_Than/1 -> OR/2
  Two_Pi_Constant/1 -> Modulus/2
  Modulus/1 -> Subtract/1
  Pi_Constant_2/1 -> Subtract/2
  OR/1 -> Select_Angle/2
  Subtract/1 -> Select_Angle/1
  Pi_Constant_1/1 -> Add/2
  Add/1 -> Modulus/1
  Difference/1 -> Select_Angle/3, Greater_Than/1, Add/1, Less_Than/1
  Select_Angle/1 -> Scale_Time/1
  Neg_Pi_Constant/1 -> Less_Than/2
  Pi_Constant_3/1 -> Greater_Than/2
  Scale_Time/1 -> velocity/1  "velocity"
  controller_mode/1 -> Terminator/1

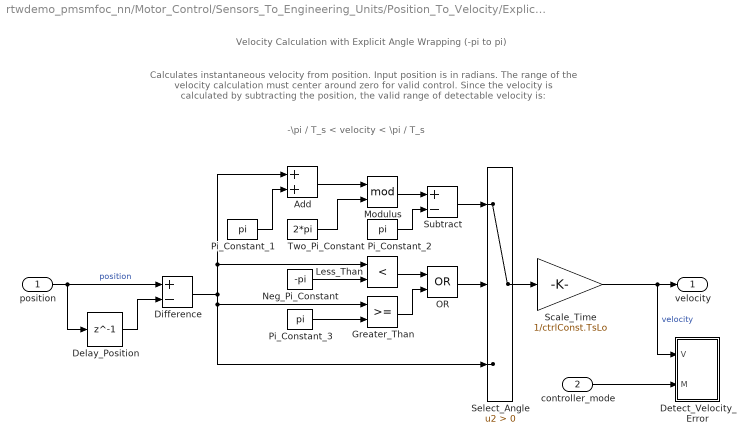
== system rtwdemo_pmsmfoc_nn/Motor_Control/Sensors_To_Engineering_Units/Position_To_Velocity/Explicit_Angle_Wrap_With_Error ==
  note: Velocity Calculation with Explicit Angle Wrapping (-pi to pi)
  note: -\pi / T_s < velocity < \pi / T_s
  note: Calculates instantaneous velocity from position. Input position is in radians.
      | The range of the velocity calculation must center around zero for valid control.
      | Since the velocity is calculated by subtracting the position, the valid range of detectable velocity is:
  position : Inport
  controller_mode : Inport  Port=2
  Add : Sum
  Delay_Position : Delay  DelayLength=1
  Detect_Velocity_Error : Subsystem
  Difference : Sum  Inputs=+-
  Greater_Than : RelationalOperator  OutDataTypeStr=boolean
  Less_Than : RelationalOperator  Operator=<  OutDataTypeStr=boolean
  Modulus : Math  Operator=mod  SaturateOnIntegerOverflow=on
  Neg_Pi_Constant : Constant  Value=-pi  OutDataTypeStr=single
  OR : Logic  Operator=OR  AllPortsSameDT=off  OutDataTypeStr=boolean
  Pi_Constant_1 : Constant  Value=pi  OutDataTypeStr=single
  Pi_Constant_2 : Constant  Value=pi  OutDataTypeStr=single
  Pi_Constant_3 : Constant  Value=pi  OutDataTypeStr=single
  Scale_Time : Gain  Gain=1/ctrlConst.TsLo  OutDataTypeStr=single
      settings: AttributesFormatString=---------------------\n%<Gain>
  Select_Angle : Switch  Criteria=u2 > Threshold
  Subtract : Sum  Inputs=+-
  Two_Pi_Constant : Constant  Value=2*pi  OutDataTypeStr=single
  velocity : Outport
  wires:
  Scale_Time/1 -> velocity/1, Detect_Velocity_Error/1(V)  "velocity"
  Pi_Constant_3/1 -> Greater_Than/2
  Neg_Pi_Constant/1 -> Less_Than/2
  Difference/1 -> Less_Than/1, Add/1, Greater_Than/1, Select_Angle/3
  Add/1 -> Modulus/1
  Pi_Constant_1/1 -> Add/2
  Subtract/1 -> Select_Angle/1
  OR/1 -> Select_Angle/2
  Pi_Constant_2/1 -> Subtract/2
  Modulus/1 -> Subtract/1
  Two_Pi_Constant/1 -> Modulus/2
  Greater_Than/1 -> OR/2
  Less_Than/1 -> OR/1
  position/1 -> Difference/1, Delay_Position/1  "position"
  Delay_Position/1 -> Difference/2
  Select_Angle/1 -> Scale_Time/1
  controller_mode/1 -> Detect_Velocity_Error/2(M)

== system rtwdemo_pmsmfoc_nn/Motor_Control/Sensors_To_Engineering_Units/Position_To_Velocity/Implicit_Integer_Wrap_With_Error ==
  note: Velocity Calculation with Scaling and Implicit
      | 32-Bit Integer Wrapping (-pi to pi)
  note: Calculates instantaneous velocity from position. Calculates instantaneous velocity from position (radians).
      | Leverages integer mathematics to handle wrapping the angle. To produce valid results, the input position must be bounded:
  note: -\pi / T_s < velocity < \pi / T_s
  note: The range of the velocity calculation must center around zero for valid control.
      | Since the velocity is calculated by subtracting the position, the valid range of detectable velocity is:
  note: -4\pi < position < 4\pi
  position : Inport  OutMin=-4*pi  OutMax=4*pi
      settings: AttributesFormatString="------------------\\nMin =  %<OutMin>\\nMax =  %<OutMax>"
  controller_mode : Inport  Port=2
  Convert_to_Uint32 : DataTypeConversion  OutDataTypeStr=int32  RndMeth=Simplest
  Detect_Velocity_Error : Subsystem
  Difference_Wrap : Sum  Inputs=+-  AccumDataTypeStr=int32  OutDataTypeStr=int32
  Difference_to_Single : DataTypeConversion  OutDataTypeStr=single
  Position_Delay : Delay  DelayLength=1
  Scale_Input : Gain  Gain=((2^31) - 1)/(4*pi)  ParamDataTypeStr=single  OutDataTypeStr=single
      settings: AttributesFormatString=---------------------------------\n%<Gain>
  Scale_Output : Gain  Gain=pi/(2^31 -1)/ctrlConst.TsLo  ParamDataTypeStr=single  OutDataTypeStr=single
      settings: AttributesFormatString=---------------------------------\n%<Gain>
  Wrap_To_Pi : Gain  Gain=4  RndMeth=Simplest  OutDataTypeStr=Inherit: Same as input  ParamDataTypeStr=Inherit: Same as input
  velocity : Outport
  wires:
  Difference_to_Single/1 -> Scale_Output/1
  Difference_Wrap/1 -> Difference_to_Single/1
  Convert_to_Uint32/1 -> Wrap_To_Pi/1
  Position_Delay/1 -> Difference_Wrap/2
  Scale_Input/1 -> Convert_to_Uint32/1
  Scale_Output/1 -> velocity/1, Detect_Velocity_Error/1(V)  "velocity"
  position/1 -> Scale_Input/1  "position"
  Wrap_To_Pi/1 -> Difference_Wrap/1, Position_Delay/1
  controller_mode/1 -> Detect_Velocity_Error/2(M)

== system rtwdemo_pmsmfoc_nn/Motor_Control/Sensors_To_Engineering_Units/Startup_Open_Loop_Control/Open Loop Position ==
  note: Open Loop Position
  note: Generate a position signal that will be used in open loop startup mode.
      | Position is incremented at a constant acceleration.
  Enable : EnablePort  StatesWhenEnabling=reset
  Integrate_To_Position : DiscreteIntegrator  InitialConditionMode=State only (most efficient)  SampleTime=-1  ICPrevOutput=DiscIntNeverNeededParam  ICPrevScaledInput=DiscIntNeverNeededParam
  Integrate_To_Velocity : DiscreteIntegrator  InitialConditionMode=State only (most efficient)  SampleTime=-1  ICPrevOutput=DiscIntNeverNeededParam  ICPrevScaledInput=DiscIntNeverNeededParam
  Startup_Acceleration_Constant : Constant  Value=ctrlParams.StartupAcceleration
  rotor_position : Outport  InitialOutput=0
      settings: AttributesFormatString=------------------------\nInitial Output: %<InitialOutput>
  wires:
  Startup_Acceleration_Constant/1 -> Integrate_To_Velocity/1
  Integrate_To_Velocity/1 -> Integrate_To_Position/1  "velocity"
  Integrate_To_Position/1 -> rotor_position/1  "position"

== system rtwdemo_pmsmfoc_nn/Motor_Control/Field_Oriented_Controller/Current_Control/Transform_Coordinates_ABC_to_dq/Clarke_Transform ==
  note: Clarke Transform
  note: Converts balanced three-phase quantities into balanced two-phase quantities.
      | The A and B phases are converted to the direct axis (alpha) component and the quadrature axis (beta) component.
      | The alpha and beta components are still dependent on time and speed.
  phase_currents : Inport
  A_phase_current : Selector  InputPortWidth=2  IndexOptions=Index vector (dialog)  Indices=1  OutputSizes=1
  Add : Sum
  B_Gain : Gain  Gain=2
  B_phase_current : Selector  InputPortWidth=2  IndexOptions=Index vector (dialog)  Indices=2  OutputSizes=1
  Beta_Gain : Gain  Gain=1/sqrt(3)
  alpha_current : Outport
  beta_current : Outport  Port=2
  wires:
  B_phase_current/1 -> B_Gain/1
  B_Gain/1 -> Add/2
  Add/1 -> Beta_Gain/1
  Beta_Gain/1 -> beta_current/1
  phase_currents/1 -> A_phase_current/1, B_phase_current/1
  A_phase_current/1 -> Add/1, alpha_current/1

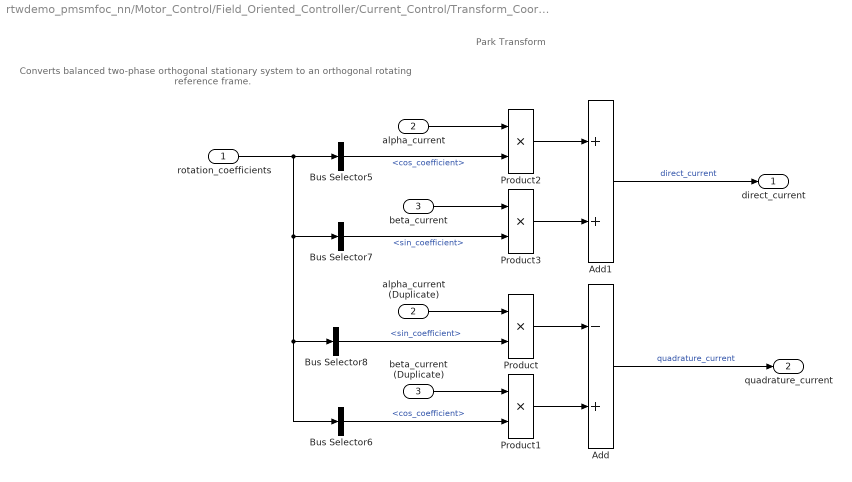
== system rtwdemo_pmsmfoc_nn/Motor_Control/Field_Oriented_Controller/Current_Control/Transform_Coordinates_ABC_to_dq/Park_Transform ==
  note: Park Transform
  note: Converts balanced two-phase orthogonal stationary system to an orthogonal rotating reference frame.
  rotation_coefficients : Inport
  alpha_current : Inport  Port=2
  beta_current : Inport  Port=3
  Add : Sum  Inputs=-+
  Add1 : Sum
  Bus Selector5 : BusSelector  OutputSignals=cos_coefficient
  Bus Selector6 : BusSelector  OutputSignals=cos_coefficient
  Bus Selector7 : BusSelector  OutputSignals=sin_coefficient
  Bus Selector8 : BusSelector  OutputSignals=sin_coefficient
  Product{,1..3} (4 alike) : Product  RndMeth=Zero
  alpha_current (Duplicate) : InportShadow  Port=2
  beta_current (Duplicate) : InportShadow  Port=3
  direct_current : Outport
  quadrature_current : Outport  Port=2
  wires:
  Product/1 -> Add/1
  Product1/1 -> Add/2
  Add/1 -> quadrature_current/1  "quadrature_current"
  Product2/1 -> Add1/1
  Product3/1 -> Add1/2
  Add1/1 -> direct_current/1  "direct_current"
  alpha_current (Duplicate)/1 -> Product/1
  Bus Selector8/1 -> Product/2  "<sin_coefficient>"
  Bus Selector6/1 -> Product1/2  "<cos_coefficient>"
  beta_current (Duplicate)/1 -> Product1/1
  alpha_current/1 -> Product2/1
  Bus Selector5/1 -> Product2/2  "<cos_coefficient>"
  beta_current/1 -> Product3/1
  Bus Selector7/1 -> Product3/2  "<sin_coefficient>"
  rotation_coefficients/1 -> Bus Selector5/1, Bus Selector7/1, Bus Selector8/1, Bus Selector6/1

== system rtwdemo_pmsmfoc_nn/Motor_Control/Field_Oriented_Controller/Current_Control/Transform_Coordinates_dq_to_ABC/Alpha_Beta_to_ABC ==
  note: 1) Only subsystems can be added as variant choices at this level
      | 2) Blocks cannot be connected at this level as connectivity is
      | automatically determined at simulation, based on the active variant
  note: Specifies which Alpha Beta to ABC coordinate transform to use.
      | The Inverse Clarke Transform is a direct sinusoidal coordinate transformation.
      | Space Vector Modulation is a technique to achieve an additional 15% increase in relative voltages between phases.
  note: Alpha Beta to ABC (Variant Subsystem)
  alpha_voltage : Inport
  beta_voltage : Inport  Port=2
  Inverse_Clarke_Transform : Subsystem  VariantObject=INVERSE_CLARKE_TRANSFORM
  Space_Vector_Modulation : Subsystem  VariantObject=SPACE_VECTOR_MODULATION
  phase_voltages : Outport

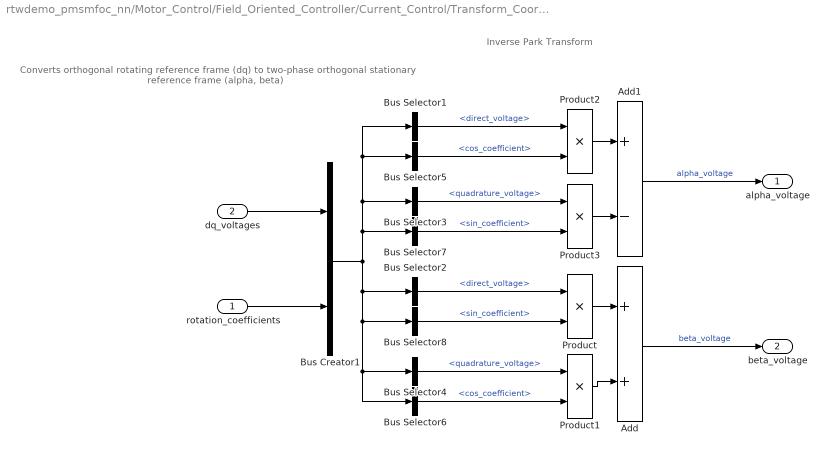
== system rtwdemo_pmsmfoc_nn/Motor_Control/Field_Oriented_Controller/Current_Control/Transform_Coordinates_dq_to_ABC/Inverse_Park_Transform ==
  note: Inverse Park Transform
  note: Converts orthogonal rotating reference frame (dq) to two-phase orthogonal stationary reference frame (alpha, beta)
  rotation_coefficients : Inport
  dq_voltages : Inport  Port=2
  Add : Sum
  Add1 : Sum  Inputs=+-
  Bus Creator1 : BusCreator  Inputs=2
  Bus Selector1 : BusSelector  OutputSignals=signal1.direct_voltage
  Bus Selector2 : BusSelector  OutputSignals=signal1.direct_voltage
  Bus Selector3 : BusSelector  OutputSignals=signal1.quadrature_voltage
  Bus Selector4 : BusSelector  OutputSignals=signal1.quadrature_voltage
  Bus Selector5 : BusSelector  OutputSignals=signal2.cos_coefficient
  Bus Selector6 : BusSelector  OutputSignals=signal2.cos_coefficient
  Bus Selector7 : BusSelector  OutputSignals=signal2.sin_coefficient
  Bus Selector8 : BusSelector  OutputSignals=signal2.sin_coefficient
  Product{,1..3} (4 alike) : Product  RndMeth=Zero
  alpha_voltage : Outport
  beta_voltage : Outport  Port=2
  wires:
  Product/1 -> Add/1
  Product1/1 -> Add/2
  Add/1 -> beta_voltage/1  "beta_voltage"
  Product2/1 -> Add1/1
  Product3/1 -> Add1/2
  Add1/1 -> alpha_voltage/1  "alpha_voltage"
  Bus Selector2/1 -> Product/1  "<direct_voltage>"
  Bus Selector8/1 -> Product/2  "<sin_coefficient>"
  Bus Selector6/1 -> Product1/2  "<cos_coefficient>"
  Bus Selector4/1 -> Product1/1  "<quadrature_voltage>"
  Bus Selector5/1 -> Product2/2  "<cos_coefficient>"
  Bus Selector3/1 -> Product3/1  "<quadrature_voltage>"
  Bus Selector7/1 -> Product3/2  "<sin_coefficient>"
  dq_voltages/1 -> Bus Creator1/1
  rotation_coefficients/1 -> Bus Creator1/2
  Bus Selector1/1 -> Product2/1  "<direct_voltage>"
  Bus Creator1/1 -> Bus Selector1/1, Bus Selector5/1, Bus Selector3/1, Bus Selector7/1, Bus Selector2/1, Bus Selector8/1, Bus Selector4/1, Bus Selector6/1

== system rtwdemo_pmsmfoc_nn/Motor_Control/Sensors_To_Engineering_Units/Position_To_Velocity/Explicit_Angle_Wrap_With_Error/Detect_Velocity_Error ==
  note: Detect Velocity Change Error
  note: If the controller is in VelocityControl mode and the velocity changes more than a realistic amount
      | then generate an error.
  V : Inport
  M : Inport  Port=2
  AND : Logic  AllPortsSameDT=off  OutDataTypeStr=boolean
  Enumerated_Constant : simulink/Sources/Enumerated Constant  OutDataTypeStr=Enum: EnumControllerMode  Value=EnumControllerMode.VelocityControl  SampleTime=inf
  Excessive_Velocity_Change : RelationalOperator  OutDataTypeStr=boolean
  Generate_Error : Subsystem  TreatAsAtomicUnit=on
  Max_Valid_Velocity_Change : Constant  Value=pi/ctrlConst.TsLo  OutDataTypeStr=single
  Relational_Operator : RelationalOperator  Operator===  OutDataTypeStr=boolean
  Velocity_Abs : Abs
  Velocity_Delay : Delay  DelayLength=1
  Velocity_Difference : Sum  Inputs=+-
  wires:
  Velocity_Abs/1 -> Excessive_Velocity_Change/1
  Max_Valid_Velocity_Change/1 -> Excessive_Velocity_Change/2
  Velocity_Difference/1 -> Velocity_Abs/1
  Velocity_Delay/1 -> Velocity_Difference/2
  V/1 -> Velocity_Difference/1, Velocity_Delay/1  "velocity"
  M/1 -> Relational_Operator/1  "controller_mode"
  Enumerated_Constant/1 -> Relational_Operator/2
  Excessive_Velocity_Change/1 -> AND/2
  Relational_Operator/1 -> AND/1
  AND/1 -> Generate_Error/Enable
